simulink model "POC_Model"  (R2017b)
settings: Solver=VariableStepAuto  StartTime=0.0  StopTime=10.0  RelTol=1e-3
values from neighbouring files (symbols this model uses):
  Amp0d = [0 0 0]    [System.m]
  Amp0n = [0 0 0]    [System.m]
  AmpSat0 = 0    [System.m]
  Elec0d = [1]    [DEFAULT.m]    (also in System.m = [0 0 0]; Trajectory.mat = [0 0 1])
  Elec0n = [1]    [DEFAULT.m]    (also in System.m = [0 0 1]; Trajectory.mat = [0 0 1])
  FB1 = 1/Sens1    [Control.m]
  Mech0d = [1]    [DEFAULT.m]    (also in System.m = [0 0 0]; Trajectory.mat = [1 102.564 2626.767504])
  Mech0n = [1]    [DEFAULT.m]    (also in System.m = [0 1 0]; Trajectory.mat = [0 0 2629.843524])
  PID0 = [0 0 0]    [Control.m]
  PID1 = [0 0 0]    [Control.m]
  TConst0 = 1    [DEFAULT.m]    (also in System.m = 0; Trajectory.mat)
undefined symbols (not defined in the file or in its folder): Amp1d, Amp1n, AmpSat1, BackEMF1, Elec1d, Elec1n, JntSat1, magnitude, Mech1d, Mech1n, Sens1, SensSat1, TConst1
libraries: simulink x7
settings Model: Creator=bowen  LastModifiedBy=bowen

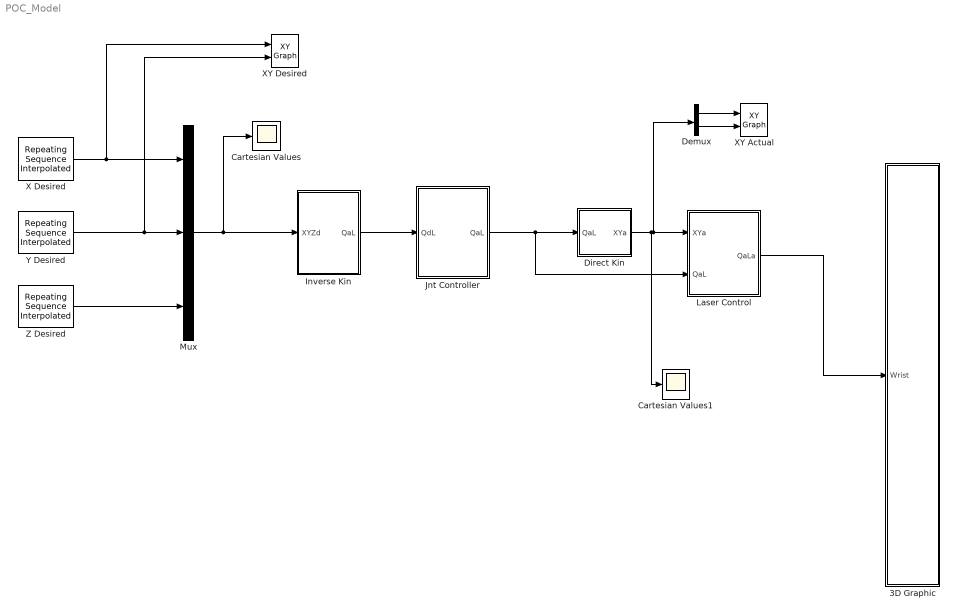
== system POC_Model ==
  3D Graphic : Subsystem
  Cartesian Values : Scope
  Cartesian Values1 : Scope
  Demux : Demux  Outputs=2
  Direct Kin : Subsystem
  Inverse Kin : Subsystem
  Jnt Controller : Subsystem
  Laser Control : Subsystem
  Mux : Mux  Inputs=3
  X Desired : simulink/Sources/Repeating Sequence Interpolated  OutValues=Xd  TimeValues=Time  LookUpMeth=Interpolation-Use End Values  tsamp=SampleTime  OutMin=[]  OutMax=[]  OutDataTypeStr=double  OutputDataTypeScalingMode=double  OutDataType=fixdt(0,8)  OutScaling=2^-10
  XY Actual : simulink/Sinks/XY Graph  xmin=-110  xmax=110  ymin=-110  ymax=110  st=-1
  XY Desired : simulink/Sinks/XY Graph  xmin=-110  xmax=110  ymin=-110  ymax=110  st=-1
  Y Desired : simulink/Sources/Repeating Sequence Interpolated  OutValues=Yd  TimeValues=Time  LookUpMeth=Interpolation-Use End Values  tsamp=SampleTime  OutMin=[]  OutMax=[]  OutDataTypeStr=double  OutputDataTypeScalingMode=double  OutDataType=fixdt(0,8)  OutScaling=2^-10
  Z Desired : simulink/Sources/Repeating Sequence Interpolated  OutValues=Zd  TimeValues=Time  LookUpMeth=Interpolation-Use End Values  tsamp=SampleTime  OutMin=[]  OutMax=[]  OutDataTypeStr=double  OutputDataTypeScalingMode=double  OutDataType=fixdt(0,8)  OutScaling=2^-10
  wires:
  Inverse Kin/1(QaL) -> Jnt Controller/1(QdL)
  Jnt Controller/1(QaL) -> Laser Control/2(QaL), Direct Kin/1(QaL)
  Laser Control/1(QaLa) -> 3D Graphic/1(Wrist)
  X Desired/1 -> XY Desired/1, Mux/1
  Y Desired/1 -> XY Desired/2, Mux/2
  Z Desired/1 -> Mux/3
  Mux/1 -> Cartesian Values/1, Inverse Kin/1(XYZd)
  Direct Kin/1(XYa) -> Cartesian Values1/1, Demux/1, Laser Control/1(XYa)
  Demux/1 -> XY Actual/1
  Demux/2 -> XY Actual/2

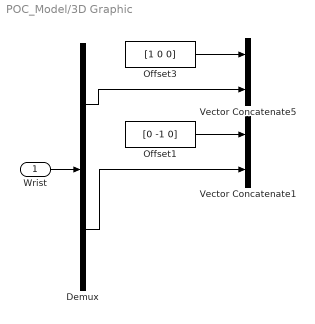
== system POC_Model/3D Graphic ==
  Wrist : Inport
  Demux : Demux  Outputs=2
  Offset1 : Constant  Value=[0 -1 0]
  Offset3 : Constant  Value=[1 0 0]
  Vector Concatenate1 : Concatenate
  Vector Concatenate5 : Concatenate
  wires:
  Demux/1 -> Vector Concatenate5/2
  Demux/2 -> Vector Concatenate1/2
  Offset3/1 -> Vector Concatenate5/1
  Offset1/1 -> Vector Concatenate1/1
  Wrist/1 -> Demux/1

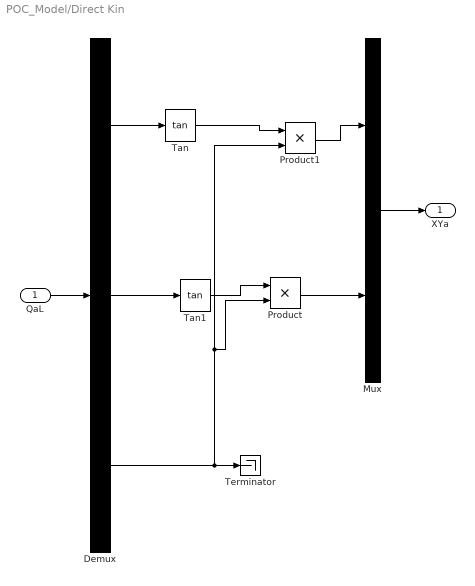
== system POC_Model/Direct Kin ==
  QaL : Inport
  Demux : Demux  Outputs=3
  Mux : Mux  Inputs=2
  Product : Product
  Product1 : Product
  Tan : Trigonometry  Operator=tan
  Tan1 : Trigonometry  Operator=tan
  Terminator : Terminator
  XYa : Outport
  wires:
  QaL/1 -> Demux/1
  Mux/1 -> XYa/1
  Demux/1 -> Tan/1
  Demux/2 -> Tan1/1
  Demux/3 -> Product/2, Product1/2, Terminator/1
  Tan/1 -> Product1/1
  Tan1/1 -> Product/1
  Product1/1 -> Mux/1
  Product/1 -> Mux/2

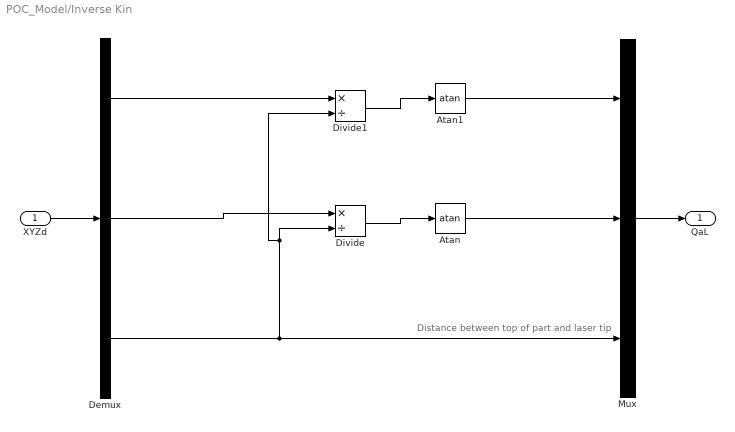
== system POC_Model/Inverse Kin ==
  note: Distance between top of part and laser tip
  XYZd : Inport
  Atan : Trigonometry  Operator=atan
  Atan1 : Trigonometry  Operator=atan
  Demux : Demux  Outputs=3
  Divide : Product  Inputs=*/
  Divide1 : Product  Inputs=*/
  Mux : Mux  Inputs=3
  QaL : Outport
  wires:
  XYZd/1 -> Demux/1
  Mux/1 -> QaL/1
  Demux/1 -> Divide1/1
  Demux/2 -> Divide/1
  Divide/1 -> Atan/1
  Atan/1 -> Mux/2
  Divide1/1 -> Atan1/1
  Atan1/1 -> Mux/1
  Demux/3 -> Divide/2, Divide1/2, Mux/3

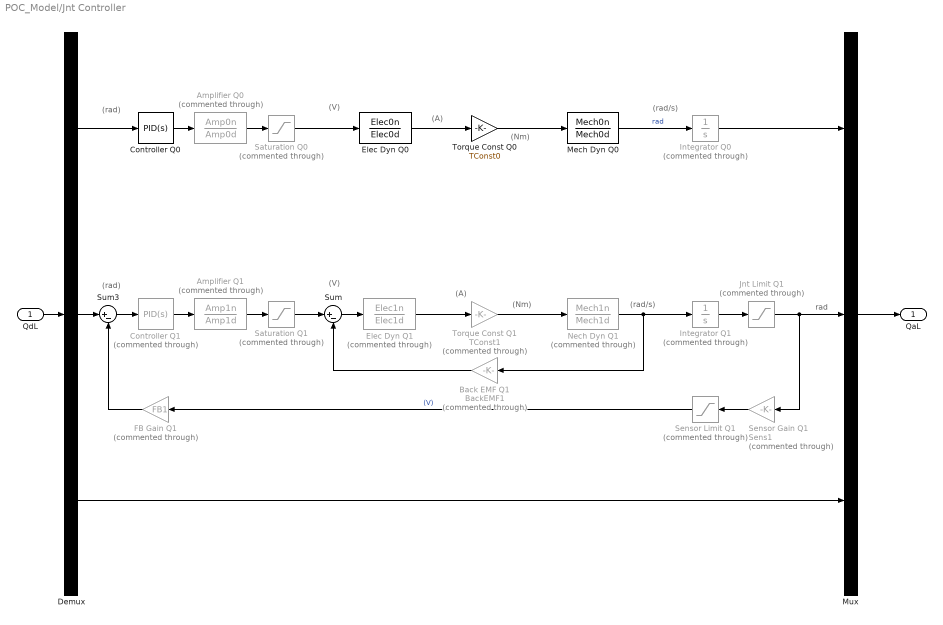
== system POC_Model/Jnt Controller ==
  note: rad
  note: (rad/s)
  note: (V)
  note: (rad)
  note: (A)
  note: (Nm)
  note: (rad/s)
  note: (V)
  note: (rad)
  note: (A)
  note: (Nm)
  QdL : Inport
  Amplifier Q0 : TransferFcn  Commented=through  Numerator=Amp0n  Denominator=Amp0d
  Amplifier Q1 : TransferFcn  Commented=through  Numerator=Amp1n  Denominator=Amp1d
  Back EMF Q1 : Gain  Commented=through  Gain=BackEMF1
  Controller Q0 : simulink/Continuous/PID Controller  Controller=PID  TimeDomain=Continuous-time  SampleTime=-1  IntegratorMethod=Forward Euler  FilterMethod=Forward Euler  Form=Parallel  UseFilter=on  ControllerParametersSource=internal  P=PID0(1)  I=PID0(2)  D=PID0(3)  N=100  InitialConditionSource=internal  InitialConditionForIntegrator=0  InitialConditionForFilter=0  ExternalReset=none  LimitOutput=off  UpperSaturationLimit=inf  LowerSaturationLimit=-inf  LinearizeAsGain=on  AntiWindupMode=none  Kb=1  TrackingMode=off  Kt=1  PParamMin=[]  PParamMax=[]  IParamMin=[]  IParamMax=[]  DParamMin=[]  DParamMax=[]  NParamMin=[]  NParamMax=[]  KbParamMin=[]  KbParamMax=[]  KtParamMin=[]  KtParamMax=[]  POutMin=[]  POutMax=[]  IOutMin=[]  IOutMax=[]  DOutMin=[]  DOutMax=[]  NOutMin=[]  NOutMax=[]  KbOutMin=[]  KbOutMax=[]  KtOutMin=[]  KtOutMax=[]  IntegratorOutMin=[]  IntegratorOutMax=[]  FilterOutMin=[]  FilterOutMax=[]  SumOutMin=[]  SumOutMax=[]  SumI1OutMin=[]  SumI1OutMax=[]  SumI2OutMin=[]  SumI2OutMax=[]  SumI3OutMin=[]  SumI3OutMax=[]  SumDOutMin=[]  SumDOutMax=[]  SaturationOutMin=[]  SaturationOutMax=[]  IntegratorContinuousStateAttributes=''  IntegratorStateMustResolveToSignalObject=off  IntegratorRTWStateStorageClass=Auto  FilterContinuousStateAttributes=''  FilterStateMustResolveToSignalObject=off  FilterRTWStateStorageClass=Auto  DifferentiatorICPrevScaledInput=0  DifferentiatorOutMin=[]  DifferentiatorOutMax=[]  InitialConditionSetting=State (most efficient)  FilterDiffOutCoefMin=[]  FilterDiffOutCoefMax=[]  SumDenOutMin=[]  SumDenOutMax=[]  SumNumOutMin=[]  SumNumOutMax=[]  ReciprocalOutMin=[]  ReciprocalOutMax=[]  DivideOutMin=[]  DivideOutMax=[]  TunerSelectOption=Transfer Function Based (PID Tuner App)
  Controller Q1 : simulink/Continuous/PID Controller  Commented=through  Controller=PID  TimeDomain=Continuous-time  SampleTime=-1  IntegratorMethod=Forward Euler  FilterMethod=Forward Euler  Form=Parallel  UseFilter=on  ControllerParametersSource=internal  P=PID1(1)  I=PID1(2)  D=PID1(3)  N=100  InitialConditionSource=internal  InitialConditionForIntegrator=0  InitialConditionForFilter=0  ExternalReset=none  LimitOutput=off  UpperSaturationLimit=inf  LowerSaturationLimit=-inf  LinearizeAsGain=on  AntiWindupMode=none  Kb=1  TrackingMode=off  Kt=1  PParamMin=[]  PParamMax=[]  IParamMin=[]  IParamMax=[]  DParamMin=[]  DParamMax=[]  NParamMin=[]  NParamMax=[]  KbParamMin=[]  KbParamMax=[]  KtParamMin=[]  KtParamMax=[]  POutMin=[]  POutMax=[]  IOutMin=[]  IOutMax=[]  DOutMin=[]  DOutMax=[]  NOutMin=[]  NOutMax=[]  KbOutMin=[]  KbOutMax=[]  KtOutMin=[]  KtOutMax=[]  IntegratorOutMin=[]  IntegratorOutMax=[]  FilterOutMin=[]  FilterOutMax=[]  SumOutMin=[]  SumOutMax=[]  SumI1OutMin=[]  SumI1OutMax=[]  SumI2OutMin=[]  SumI2OutMax=[]  SumI3OutMin=[]  SumI3OutMax=[]  SumDOutMin=[]  SumDOutMax=[]  SaturationOutMin=[]  SaturationOutMax=[]  IntegratorContinuousStateAttributes=''  IntegratorStateMustResolveToSignalObject=off  IntegratorRTWStateStorageClass=Auto  FilterContinuousStateAttributes=''  FilterStateMustResolveToSignalObject=off  FilterRTWStateStorageClass=Auto  DifferentiatorICPrevScaledInput=0  DifferentiatorOutMin=[]  DifferentiatorOutMax=[]  InitialConditionSetting=State (most efficient)  FilterDiffOutCoefMin=[]  FilterDiffOutCoefMax=[]  SumDenOutMin=[]  SumDenOutMax=[]  SumNumOutMin=[]  SumNumOutMax=[]  ReciprocalOutMin=[]  ReciprocalOutMax=[]  DivideOutMin=[]  DivideOutMax=[]  TunerSelectOption=Transfer Function Based (PID Tuner App)
  Demux : Demux  Outputs=3
  Elec Dyn Q0 : TransferFcn  Numerator=Elec0n  Denominator=Elec0d
  Elec Dyn Q1 : TransferFcn  Commented=through  Numerator=Elec1n  Denominator=Elec1d
  FB Gain Q1 : Gain  Commented=through  Gain=FB1
  Integrator Q0 : Integrator  Commented=through
  Integrator Q1 : Integrator  Commented=through
  Jnt Limit Q1 : Saturate  Commented=through  UpperLimit=JntSat1  LowerLimit=-JntSat1
  Mech Dyn Q0 : TransferFcn  Numerator=Mech0n  Denominator=Mech0d
  Mux : Mux  Inputs=3
  Nech Dyn Q1 : TransferFcn  Commented=through  Numerator=Mech1n  Denominator=Mech1d
  Saturation Q0 : Saturate  Commented=through  UpperLimit=AmpSat0  LowerLimit=-AmpSat0
  Saturation Q1 : Saturate  Commented=through  UpperLimit=AmpSat1  LowerLimit=-AmpSat1
  Sensor Gain Q1 : Gain  Commented=through  Gain=Sens1
  Sensor Limit Q1 : Saturate  Commented=through  UpperLimit=SensSat1  LowerLimit=-SensSat1
  Sum : Sum  Inputs=|+-
  Sum3 : Sum  Inputs=|+-
  Torque Const Q0 : Gain  Gain=TConst0
  Torque Const Q1 : Gain  Commented=through  Gain=TConst1
  QaL : Outport
  wires:
  QdL/1 -> Demux/1
  Mux/1 -> QaL/1
  Controller Q1/1 -> Amplifier Q1/1
  Sum/1 -> Elec Dyn Q1/1
  Sum3/1 -> Controller Q1/1
  Elec Dyn Q1/1 -> Torque Const Q1/1
  Amplifier Q1/1 -> Saturation Q1/1
  Saturation Q1/1 -> Sum/1
  Back EMF Q1/1 -> Sum/2
  Sensor Gain Q1/1 -> Sensor Limit Q1/1
  Controller Q0/1 -> Amplifier Q0/1
  Saturation Q0/1 -> Elec Dyn Q0/1
  Demux/1 -> Controller Q0/1
  Elec Dyn Q0/1 -> Torque Const Q0/1
  Amplifier Q0/1 -> Saturation Q0/1
  Torque Const Q0/1 -> Mech Dyn Q0/1
  Jnt Limit Q1/1 -> Mux/2, Sensor Gain Q1/1
  Demux/3 -> Mux/3
  Demux/2 -> Sum3/1
  FB Gain Q1/1 -> Sum3/2
  Torque Const Q1/1 -> Nech Dyn Q1/1
  Sensor Limit Q1/1 -> FB Gain Q1/1  "(V)"
  Mech Dyn Q0/1 -> Integrator Q0/1  "rad"
  Integrator Q0/1 -> Mux/1
  Integrator Q1/1 -> Jnt Limit Q1/1
  Nech Dyn Q1/1 -> Integrator Q1/1, Back EMF Q1/1

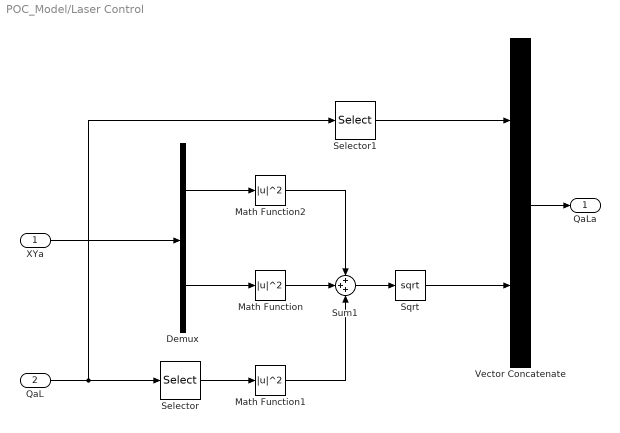
== system POC_Model/Laser Control ==
  XYa : Inport
  QaL : Inport  Port=2
  Demux : Demux  Outputs=2
  Math Function : Math  Operator=magnitude^2  SaturateOnIntegerOverflow=on
  Math Function1 : Math  Operator=magnitude^2  SaturateOnIntegerOverflow=on
  Math Function2 : Math  Operator=magnitude^2  SaturateOnIntegerOverflow=on
  Selector : Selector  InputPortWidth=3  IndexOptions=Index vector (dialog)  Indices=3  OutputSizes=1
  Selector1 : Selector  InputPortWidth=3  IndexOptions=Index vector (dialog)  Indices=[1 2]  OutputSizes=1
  Sqrt : Sqrt  SaturateOnIntegerOverflow=on
  Sum1 : Sum  Inputs=+++
  Vector Concatenate : Concatenate
  QaLa : Outport
  wires:
  Demux/2 -> Math Function/1
  Demux/1 -> Math Function2/1
  Sqrt/1 -> Vector Concatenate/2
  Math Function2/1 -> Sum1/1
  Math Function/1 -> Sum1/2
  Math Function1/1 -> Sum1/3
  Sum1/1 -> Sqrt/1
  QaL/1 -> Selector1/1, Selector/1
  XYa/1 -> Demux/1
  Selector/1 -> Math Function1/1
  Selector1/1 -> Vector Concatenate/1
  Vector Concatenate/1 -> QaLa/1
